simulink model "template"  (Simulink 9.0)
settings: Solver=FixedStepDiscrete  StartTime=0.0  StopTime=N*Ts+Ntransient  FixedStep=Ts  MaxStep=3.90625e-06  RelTol=1e-3  AbsTol=1e-3
undefined symbols (not defined in the file): argo, b, clock, Cs, delta, Fs, k, N, NCOMPARATORI, R, Ts
libraries: SDtoolbox x9
CloseFcn:
  | ;slview('closediagram',bdroot);
settings Model: SuppressorTable=22 serialization::archive 11 0 6 0 0 0 11 0  Creator=piero  ExtModeAutoUpdateStatusClock=off
settings DataIOCC: SignalLoggingSaveFormat=ModelDataLogs  SaveOutput=off  SaveTime=off  SignalLoggingName=sigsOut
settings OptimizationCC: BooleanDataType=off  InitFltsAndDblsToZero=on
settings DebuggingCC: SaveWithParameterizedLinksMsg=none  SignalResolutionControl=TryResolveAllWithWarning  MultiTaskDSMMsg=warning  MultiTaskCondExecSysMsg=none  FcnCallInpInsideContextMsg=warning  StrictBusMsg=None
settings HardwareCC: TargetUnknown=on
settings RTWCC: TemplateMakefile=grt.tmf
settings GRTTargetCC: TargetFcnLib=ansi_tfl_tmw.mat  CombineOutputUpdateFcns=off  GRTInterface=on

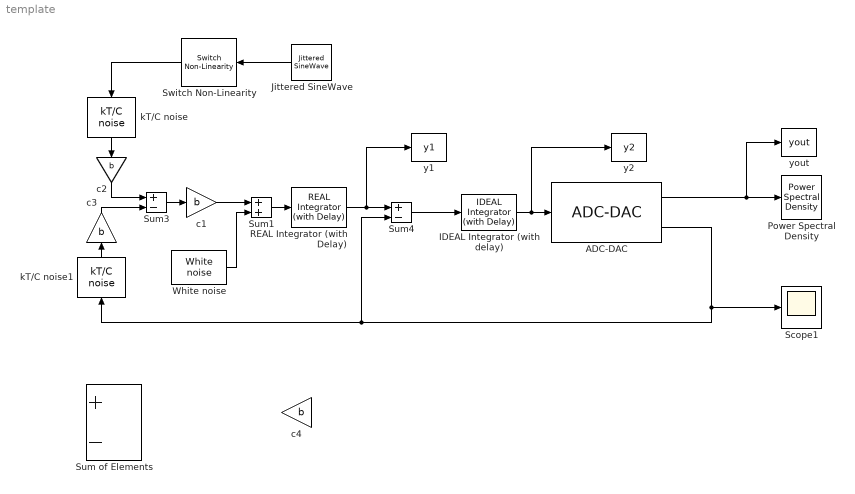
== system template ==
  " ADC-DAC" : SDtoolbox/ADC-DAC  k=NCOMPARATORI  MM=off  match=match  CST=Cs  VVG=off  argo=argo(:,3)  LF=off  NF=retA.log
  IDEAL Integrator (with delay) : SDtoolbox/IDEAL Integrator (with Delay)  Amax=Amax  Ts=Ts
  Jittered SineWave : SDtoolbox/Jittered SineWave  Ampl=Ampl  Bias=0  Freq=finrad  Phase=0  SampJ=delta*0  Ts=Ts  seed=floor(100*sum(clock))
  Power Spectral Density : SDtoolbox/Power Spectral Density  SN=1  Fs=Fs  fBL=1  fBH=Fs/(2*R)  Fin=Fin  N=N  Ntransient=Ntransient  VW=off  savename=savemat  Scale_type=logarithmic
  REAL Integrator (with Delay) : SDtoolbox/REAL Integrator (with Delay)  Ts=Ts  alfa=alfa  Amax=Amax  sr=sr  GBW=GBW
  Scope1 : Scope
  Sum of Elements : Sum  Inputs=+-
  Sum1 : Sum  SaturateOnIntegerOverflow=on  InputSameDT=on  OutDataTypeStr=Inherit: Same as first input
  Sum3 : Sum  Inputs=+-  SaturateOnIntegerOverflow=on  InputSameDT=on  OutDataTypeStr=Inherit: Same as first input
  Sum4 : Sum  Inputs=+-  SaturateOnIntegerOverflow=on  InputSameDT=on  OutDataTypeStr=Inherit: Same as first input
  Switch Non-Linearity : SDtoolbox/Switch Non-Linearity  Ts=Ts  CS=Cs  VsupplyP=2  VsupplyN=-2  Size=20  KPN=175e-6  KPP=60e-6  VTN=0.5  VTP=-0.5  BS=0
  White noise : SDtoolbox/White noise  seed=floor(sum(clock)^1/111)  Ts=Ts  noise=noise1
  c{1..4} (4 alike) : Gain  Gain=b  SaturateOnIntegerOverflow=on  OutDataTypeStr=Inherit: Same as input  ParamDataTypeStr=Inherit: Same as input
  kT/C noise : SDtoolbox/kT//C noise  Ts=Ts  C=Cs  Temp=Temp  k=k  seed=floor(sum(clock))
  kT/C noise1 : SDtoolbox/kT//C noise  Ts=Ts  C=Cs  Temp=Temp  k=k  seed=floor(sum(clock))
  y1 : ToWorkspace  VariableName=y1  SampleTime=-1
  y2 : ToWorkspace  VariableName=y2  SampleTime=-1
  yout : ToWorkspace  VariableName=yout  SampleTime=-1
  wires:
  Sum4/1 -> IDEAL Integrator (with delay)/1
  Sum3/1 -> c1/1
  " ADC-DAC"/2 -> Scope1/1, Sum4/2, kT/C noise1/1
  c1/1 -> Sum1/1
  kT/C noise/1 -> c2/1
  White noise/1 -> Sum1/2
  " ADC-DAC"/1 -> Power Spectral Density/1, yout/1
  IDEAL Integrator (with delay)/1 -> y2/1, " ADC-DAC"/1
  Jittered SineWave/1 -> Switch Non-Linearity/1
  c2/1 -> Sum3/1
  c3/1 -> Sum3/2
  kT/C noise1/1 -> c3/1
  Sum1/1 -> REAL Integrator (with Delay)/1
  REAL Integrator (with Delay)/1 -> Sum4/1, y1/1
  Switch Non-Linearity/1 -> kT/C noise/1
